simulink model "Copy_of_simpleDemonstrationDouble"  (R2023a)
settings: Solver=VariableStepAuto  StartTime=0.0  StopTime=Tstep*ofdmSymLen*6  RelTol=1e-3
PreLoadFcn:
  | % 100 MHz scenario
  | scs = 30e3;
  | fftLength = 4096;
  | NSubcarriers = 3276;
  | cpLength = 288;
  | windowLength = 20;
  | 
  | nGuardBandCarrier = fftLength - NSubcarriers;
  | ofdmSymLen = fftLength+cpLength;
  | overSamplingRate = 7;
  | filterLength = 6*70;
  | 
  | BW = scs*fftLength;                       %  Signal BW
  | Tstep = 1/BW;                   %  Simulation BW BB
  | RF = 3.7e9;                       %  RF center frequency
  | IF = 500e6;                          % IF frequency
  | dataRatePA = 1/BW;  % PA characterization sample time
  | N = nGuardBandCarrier/2;
  | HPF_cutoff = RF - 500e6;
  | 
  | bw = 100e6;
  | [txWaveform, sampleRate] = helperPACharGenerateOFDM(bw);
  | 
  | dataFileName = sprintf("helperPACharSavedData%dMHz",bw/1e6);
  | load(dataFileName,"results")
  | paInput = results.InputWaveform;
  | paOutput = results.OutputWaveform;
  | modType = 'memPoly';
  | memLen = 5;
  | degLen = 5;
  | halfDataPts = round(length(paInput)/2);
  | origState = warning;
  | warning('off', 'MATLAB:rankDeficientMatrix')
  | paModelMemPoly = double(helperPACharMemPolyModel('coefficientFinder', ...
  |   paInput(1:halfDataPts),paOutput(1:halfDataPts),memLen,degLen,modType));
  | warning(origState);
  | 
  | gain = results.LinearGain;
  | scaleFactor = double(max(abs(paOutput))/max(abs(txWaveform))/gain);
InitFcn:
  | % Initialize model parameters
  | NRInfo = get_param([gcs '/5G NR Test Model'], 'UserData');
  | MultirateBlock = [gcs '/Multirate Parameters'];
  | hInitializeNRTMModel(MultirateBlock,NRInfo);
StopFcn:
  | clear hDecodeSubframe;
undefined symbols (not defined in the file or in its folder): errorPDec, errorPInt, errorStDec, errorStInt, firceqrip, modNFloor, nDec, nInt, OSR, Probability, S, waveform
libraries: simrfV2elements x20, simrfV2util1 x11, simrfV2_lib x5, dspstat3 x4, simrfV2systems x3, commofdm x2, commrfcorlib x2, dspmlti4 x2, simrfV2junction1 x2, commrandsrc3 x1, commdigbbndam3 x1, commutil2 x1
(part 2 of 2)

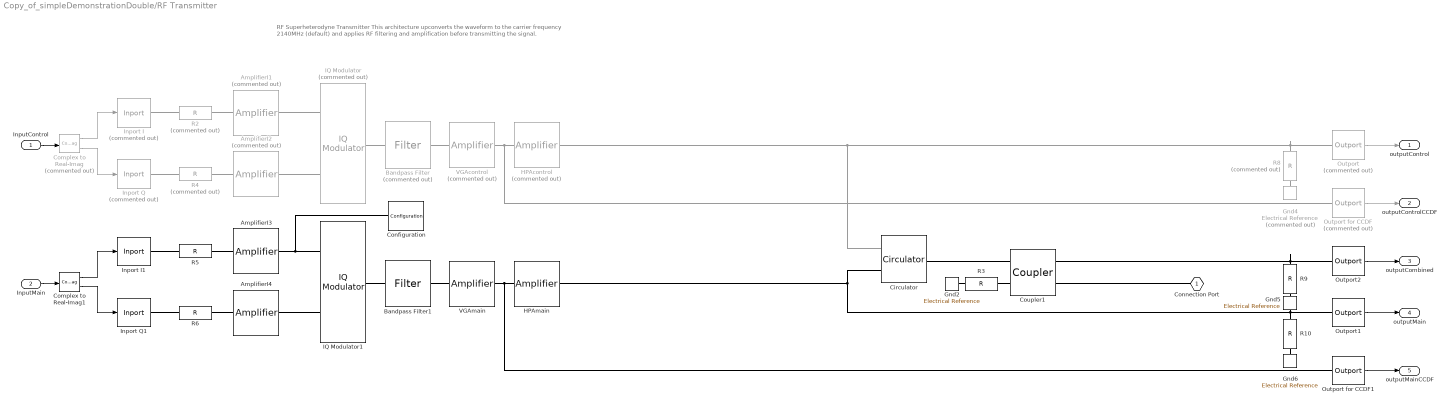
== system Copy_of_simpleDemonstrationDouble/RF Transmitter ==
  note: RF Superheterodyne Transmitter
      |
      | This architecture upconverts the waveform to the carrier frequency 2140MHz (default) and applies RF
      | filtering and amplification before transmitting the signal.
  InputControl : Inport
  InputMain : Inport  Port=2
  AmplifierI1 : simrfV2elements/Amplifier  Commented=on  classname=amplifier  DataSource=Data file  File=unitygain.s2p  isNetworkObj=off  Paramtype=S-parameters  Sparam=[0 0;1 0]  SparamFreq=1e9 Hz  SparamZ0=50  isRationalObj=off  Residues=0  Poles=0  DF={0 0; 1 0}  Source_linear_gain=Available power gain  linear_gain=10*log10(4) dB  AmAmAmPmTable=[-25,5,-1;-10,20,-2;0,27,5;5,28,12]  Zin=50  Zout=50  Source_Poly=Even and odd order  Poly_Coeffs=[0 1]  IPType=Input  IP2=inf dBm  IP3=inf dBm  P1dB=inf dBm  Psat=inf dBm  Gcomp=inf dBm  InternalGrounding=on  SourceFreq=Extracted from data source  PlotFreq=[1e9:1e6:3e9] Hz  PlotType=X-Y plane  YParam1=S(1,1)  YFormat1=Magnitude (dB)  YParam2=None  YFormat2=Magnitude (dB)  YOption=Linear  XOption=Linear  SparamRepresentation=Time domain (rationalfit)  FitTol=-40  FitOpt=Fit individually  MaxPoles=48  AutoImpulseLength=on  ImpulseLength=1e-10 s  MagModeling=off  AddNoise=on  NoiseType=Noise figure  NoiseDist=White  NF=0.2  MinNF=0  Gopt=0  RN=0  CarrierFreq=0 Hz  NoiseAutoImpulseLength=on  NoiseImpulseLength=1e-10 s  ConstS21NL=on  OpFreq=0 Hz  SetOpFreqAsMaxS21=on
  AmplifierI2 : simrfV2elements/Amplifier  Commented=on  classname=amplifier  DataSource=Data file  File=unitygain.s2p  isNetworkObj=off  Paramtype=S-parameters  Sparam=[0 0;1 0]  SparamFreq=1e9 Hz  SparamZ0=50  isRationalObj=off  Residues=0  Poles=0  DF={0 0; 1 0}  Source_linear_gain=Available power gain  linear_gain=10*log10(4) dB  AmAmAmPmTable=[-25,5,-1;-10,20,-2;0,27,5;5,28,12]  Zin=50  Zout=50  Source_Poly=Even and odd order  Poly_Coeffs=[0 1]  IPType=Input  IP2=inf dBm  IP3=inf dBm  P1dB=inf dBm  Psat=inf dBm  Gcomp=inf dBm  InternalGrounding=on  SourceFreq=Extracted from data source  PlotFreq=[1e9:1e6:3e9] Hz  PlotType=X-Y plane  YParam1=S(1,1)  YFormat1=Magnitude (dB)  YParam2=None  YFormat2=Magnitude (dB)  YOption=Linear  XOption=Linear  SparamRepresentation=Time domain (rationalfit)  FitTol=-40  FitOpt=Fit individually  MaxPoles=48  AutoImpulseLength=on  ImpulseLength=1e-10 s  MagModeling=off  AddNoise=on  NoiseType=Noise figure  NoiseDist=White  NF=0.2  MinNF=0  Gopt=0  RN=0  CarrierFreq=0 Hz  NoiseAutoImpulseLength=on  NoiseImpulseLength=1e-10 s  ConstS21NL=on  OpFreq=0 Hz  SetOpFreqAsMaxS21=on
  AmplifierI3 : simrfV2elements/Amplifier  classname=amplifier  DataSource=Data file  File=unitygain.s2p  isNetworkObj=off  Paramtype=S-parameters  Sparam=[0 0;1 0]  SparamFreq=1e9 Hz  SparamZ0=50  isRationalObj=off  Residues=0  Poles=0  DF={0 0; 1 0}  Source_linear_gain=Available power gain  linear_gain=10*log10(4) dB  AmAmAmPmTable=[-25,5,-1;-10,20,-2;0,27,5;5,28,12]  Zin=50  Zout=50  Source_Poly=Even and odd order  Poly_Coeffs=[0 1]  IPType=Input  IP2=inf dBm  IP3=inf dBm  P1dB=inf dBm  Psat=inf dBm  Gcomp=inf dBm  InternalGrounding=on  SourceFreq=Extracted from data source  PlotFreq=[1e9:1e6:3e9] Hz  PlotType=X-Y plane  YParam1=S(1,1)  YFormat1=Magnitude (dB)  YParam2=None  YFormat2=Magnitude (dB)  YOption=Linear  XOption=Linear  SparamRepresentation=Time domain (rationalfit)  FitTol=-40  FitOpt=Fit individually  MaxPoles=48  AutoImpulseLength=on  ImpulseLength=1e-10 s  MagModeling=off  AddNoise=on  NoiseType=Noise figure  NoiseDist=White  NF=0.2  MinNF=0  Gopt=0  RN=0  CarrierFreq=0 Hz  NoiseAutoImpulseLength=on  NoiseImpulseLength=1e-10 s  ConstS21NL=on  OpFreq=0 Hz  SetOpFreqAsMaxS21=on
  AmplifierI4 : simrfV2elements/Amplifier  classname=amplifier  DataSource=Data file  File=unitygain.s2p  isNetworkObj=off  Paramtype=S-parameters  Sparam=[0 0;1 0]  SparamFreq=1e9 Hz  SparamZ0=50  isRationalObj=off  Residues=0  Poles=0  DF={0 0; 1 0}  Source_linear_gain=Available power gain  linear_gain=10*log10(4) dB  AmAmAmPmTable=[-25,5,-1;-10,20,-2;0,27,5;5,28,12]  Zin=50  Zout=50  Source_Poly=Even and odd order  Poly_Coeffs=[0 1]  IPType=Input  IP2=inf dBm  IP3=inf dBm  P1dB=inf dBm  Psat=inf dBm  Gcomp=inf dBm  InternalGrounding=on  SourceFreq=Extracted from data source  PlotFreq=[1e9:1e6:3e9] Hz  PlotType=X-Y plane  YParam1=S(1,1)  YFormat1=Magnitude (dB)  YParam2=None  YFormat2=Magnitude (dB)  YOption=Linear  XOption=Linear  SparamRepresentation=Time domain (rationalfit)  FitTol=-40  FitOpt=Fit individually  MaxPoles=48  AutoImpulseLength=on  ImpulseLength=1e-10 s  MagModeling=off  AddNoise=on  NoiseType=Noise figure  NoiseDist=White  NF=0.2  MinNF=0  Gopt=0  RN=0  CarrierFreq=0 Hz  NoiseAutoImpulseLength=on  NoiseImpulseLength=1e-10 s  ConstS21NL=on  OpFreq=0 Hz  SetOpFreqAsMaxS21=on
  Bandpass Filter : simrfV2elements/Filter  Commented=on  classname=filter  DesignMethod=Chebyshev  ResponseType=Bandpass  Implementation=Transfer function  ImplementationIdeal=Constant per carrier  ImplementationRational=Transfer function  UseFilterOrder=off  FilterOrder=5  PassFreq_lp=1 GHz  PassFreq_hp=2 GHz  PassFreq_bp=bpFilterPassFreq MHz  PassFreq_bs=[1 4] GHz  PassAtten=bpFilterPassAtten  StopFreq_lp=2 GHz  StopFreq_hp=1 GHz  StopFreq_bp=bpFilterStopFreq MHz  StopFreq_bs=[2.1 2.9] GHz  StopAtten=bpFilterStopAtten  Rsrc=bpFilterImpedance  Rload=bpFilterImpedance  AutoImpulseLength=on  ImpulseLength=1e-10 s  InternalGrounding=on  PlotFuncLeft=Voltage transfer  PlotLeftForm=Magnitude (dB)  PlotRightOnVT=None  PlotRightNoTD=None  PlotRightNoGD=None  PlotRightNoIR=None  PlotRightNoSR=None  PlotRightForm=Magnitude (dB)  FreqPoints=logspace(0,10,101)  Freq_unit=Hz  TimePoints=linspace(0,1,1e6+1)  Time_unit=s  XaxisScale=Linear  YaxisScale=Linear  needRedraw=1
  Bandpass Filter1 : simrfV2elements/Filter  classname=filter  DesignMethod=Chebyshev  ResponseType=Bandpass  Implementation=Transfer function  ImplementationIdeal=Constant per carrier  ImplementationRational=Transfer function  UseFilterOrder=off  FilterOrder=5  PassFreq_lp=1 GHz  PassFreq_hp=2 GHz  PassFreq_bp=bpFilterPassFreq MHz  PassFreq_bs=[1 4] GHz  PassAtten=bpFilterPassAtten  StopFreq_lp=2 GHz  StopFreq_hp=1 GHz  StopFreq_bp=bpFilterStopFreq MHz  StopFreq_bs=[2.1 2.9] GHz  StopAtten=bpFilterStopAtten  Rsrc=bpFilterImpedance  Rload=bpFilterImpedance  AutoImpulseLength=on  ImpulseLength=1e-10 s  InternalGrounding=on  PlotFuncLeft=Voltage transfer  PlotLeftForm=Magnitude (dB)  PlotRightOnVT=None  PlotRightNoTD=None  PlotRightNoGD=None  PlotRightNoIR=None  PlotRightNoSR=None  PlotRightForm=Magnitude (dB)  FreqPoints=logspace(0,10,101)  Freq_unit=Hz  TimePoints=linspace(0,1,1e6+1)  Time_unit=s  XaxisScale=Linear  YaxisScale=Linear  needRedraw=1
  Circulator : simrfV2junction1/Circulator  classname=circulators  DataSource=Network-parameters  NumPorts=3  DeviceCirculator=Circulator counter clockwise  DeviceDivider=T power divider  DeviceCoupler=Directional coupler  Paramtype=S-parameters  Sparam=[0 0 1; 1 0 0; 0 1 0]  SparamFreq=1e9 Hz  SparamZ0=50  Phase12=0  Phase33=0  Alpha=0  NumberDividerOutports=2  Coupling=0  Directivity=inf  InsertionLoss=inf  ReturnLoss=inf  InternalGrounding=on  SparamRepresentation=Frequency domain  FitOpt=Share all poles  FitTol=-40  MaxPoles=48
  Complex to Real-Imag : ComplexToRealImag  Commented=on
  Complex to Real-Imag1 : ComplexToRealImag
  Configuration : simrfV2util1/Configuration  AutoFreq=on  Tones="[0.07        2.07] GHz"  Harmonics="[1  3]"  NormalizeCarrierPower=on  SolverType=Auto  UseCCode=on  StepSize=Tstep/overSamplingRate s  AddNoise=on  defaultRNG=on  Seed=0  Temperature=temperature K  SolverDelFlag=0  AbsTol=1e-6  RelTol=1e-3  MaxIter=10  ErrorEstimationType=2-norm over all variables  EnableInterpFilter=off  HiddenFIRfilterControllerParam=off  SmallSignalApprox=off  AllSimFreqs=on  SimFreqs=[] Hz  SimFreqsInternal=[]  SamplesPerFrame=1
  Coupler1 : simrfV2junction1/Coupler  classname=couplers  DataSource=Network-parameters  NumPorts=4  DeviceCirculator=Circulator clockwise  DeviceDivider=T power divider  DeviceCoupler=Directional coupler  Paramtype=S-parameters  Sparam=[0 0 1; 1 0 0; 0 1 0]  SparamFreq=1e9 Hz  SparamZ0=50  Phase12=0  Phase33=0  Alpha=0  NumberDividerOutports=2  Coupling=55  Directivity=inf  InsertionLoss=0.0001  ReturnLoss=inf  InternalGrounding=on  SparamRepresentation=Frequency domain  FitOpt=Share all poles  FitTol=-40  MaxPoles=48
  Gnd2 : simrfV2_lib/Elements/Electrical Reference
      settings: InternalSimscapePortConfiguration="{\"Bottom\":[],\"Left\":[{\"id\":\"V\",\"label\":\"\",\"type\":\"foundation.rf.circuitenvelope\"}],\"Right\":[],\"Top\":[]}"
  Gnd4 : simrfV2_lib/Elements/Electrical Reference  Commented=on
      settings: InternalSimscapePortConfiguration="{\"Bottom\":[],\"Left\":[{\"id\":\"V\",\"label\":\"\",\"type\":\"foundation.rf.circuitenvelope\"}],\"Right\":[],\"Top\":[]}"
  Gnd5 : simrfV2_lib/Elements/Electrical Reference
      settings: InternalSimscapePortConfiguration="{\"Bottom\":[],\"Left\":[{\"id\":\"V\",\"label\":\"\",\"type\":\"foundation.rf.circuitenvelope\"}],\"Right\":[],\"Top\":[]}"
  Gnd6 : simrfV2_lib/Elements/Electrical Reference
      settings: InternalSimscapePortConfiguration="{\"Bottom\":[],\"Left\":[{\"id\":\"V\",\"label\":\"\",\"type\":\"foundation.rf.circuitenvelope\"}],\"Right\":[],\"Top\":[]}"
  HPAcontrol : simrfV2elements/Amplifier  Commented=on  classname=amplifier  DataSource=Network-parameters  File=unitygain.s2p  isNetworkObj=off  Paramtype=S-parameters  Sparam=0  SparamFreq=CarrierFreq GHz  SparamZ0=50  isRationalObj=off  Residues=0  Poles=0  DF={0 0; 1 0}  Source_linear_gain=Available power gain  linear_gain=hpaGain - 3.5 dB  AmAmAmPmTable=[-25,5,-1;-10,20,-2;0,27,5;5,28,12]  Zin=hpaImpedance  Zout=hpaImpedance  Source_Poly=Odd order  Poly_Coeffs=[0 1]  IPType=Output  IP2=inf dBm  IP3=hpaIP3 dBm  P1dB=hpaP1dB dBm  Psat=inf dBm  Gcomp=inf dBm  InternalGrounding=on  SourceFreq=Extracted from data source  PlotFreq=1 Hz  PlotType=X-Y plane  YParam1=S(2,1)  YFormat1=Magnitude (dB)  YParam2=None  YFormat2=Magnitude (dB)  YOption=Linear  XOption=Linear  SparamRepresentation=Frequency domain  FitTol=-40  FitOpt=Fit individually  MaxPoles=48  AutoImpulseLength=off  ImpulseLength=0 s  MagModeling=off  AddNoise=on  NoiseType=Noise figure  NoiseDist=White  NF=hpaNF  MinNF=0  Gopt=0  RN=0  CarrierFreq=0 Hz  NoiseAutoImpulseLength=on  NoiseImpulseLength=1e-10 s  ConstS21NL=on  OpFreq=0 Hz  SetOpFreqAsMaxS21=on
  HPAmain : simrfV2elements/Amplifier  classname=amplifier  DataSource=Network-parameters  File=unitygain.s2p  isNetworkObj=off  Paramtype=S-parameters  Sparam=0  SparamFreq=CarrierFreq GHz  SparamZ0=50  isRationalObj=off  Residues=0  Poles=0  DF={0 0; 1 0}  Source_linear_gain=Available power gain  linear_gain=hpaGain dB  AmAmAmPmTable=[-25,5,-1;-10,20,-2;0,27,5;5,28,12]  Zin=hpaImpedance  Zout=hpaImpedance  Source_Poly=Odd order  Poly_Coeffs=[0 1]  IPType=Output  IP2=inf dBm  IP3=hpaIP3 dBm  P1dB=hpaP1dB dBm  Psat=inf dBm  Gcomp=inf dBm  InternalGrounding=on  SourceFreq=Extracted from data source  PlotFreq=1 Hz  PlotType=X-Y plane  YParam1=S(2,1)  YFormat1=Magnitude (dB)  YParam2=None  YFormat2=Magnitude (dB)  YOption=Linear  XOption=Linear  SparamRepresentation=Frequency domain  FitTol=-40  FitOpt=Fit individually  MaxPoles=48  AutoImpulseLength=off  ImpulseLength=0 s  MagModeling=off  AddNoise=on  NoiseType=Noise figure  NoiseDist=White  NF=hpaNF  MinNF=0  Gopt=0  RN=0  CarrierFreq=0 Hz  NoiseAutoImpulseLength=on  NoiseImpulseLength=1e-10 s  ConstS21NL=on  OpFreq=0 Hz  SetOpFreqAsMaxS21=on
  IQ Modulator : simrfV2systems/IQ Modulator  Commented=on  classname=iqmod  Source_linear_gain=Available power gain  linear_gain=modGain dB  Poly_Coeffs=[0 1]  LOFreq=loFreq MHz  Zin=modImpedance  Zout=modImpedance  AddIRFilters=off  AddCSFilter=off  InternalGrounding=on  ForceNextInit=off  NFloor=modNFloor  GainMismatch=modGainMismatch dB  PhaseMismatch=modPhaseMismatch deg  Isolation=modIsolation dB  AddPhaseNoise=on  PhaseNoiseOffset=modPNOffset  PhaseNoiseLevel=modPNLevel  AutoImpulseLengthPN=off  ImpulseLengthPN=impulseDuration  ImpulseLength_unitPN=s  Source_Poly=Odd order  IPType=Input  IP2=inf dBm  IP3=modIP3 dBm  P1dB=inf dBm  Psat=inf dBm  Gcomp=inf dBm  DesignMethodIR=Ideal  ResponseTypeIR=Lowpass  ImplementationIR=LC Tee  ImplementationIdealIR=Constant per carrier  ImplementationRationalIR=Transfer function  UseFilterOrderIR=on  FilterOrderIR=3  PassFreq_lpIR=1  PassFreq_lp_unitIR=GHz  PassFreq_hpIR=2  PassFreq_hp_unitIR=GHz  PassFreq_bpIR=[2 3]  PassFreq_bp_unitIR=GHz  PassFreq_bsIR=[1 4]  PassFreq_bs_unitIR=GHz  PassAttenIR=10*log10(2)  StopFreq_lpIR=2  StopFreq_lp_unitIR=GHz  StopFreq_hpIR=1  StopFreq_hp_unitIR=GHz  StopFreq_bpIR=[1.5 3.5]  StopFreq_bp_unitIR=GHz  StopFreq_bsIR=[2.1 2.9]  StopFreq_bs_unitIR=GHz  StopAttenIR=40  RsrcIR=50  RloadIR=50  AutoImpulseLengthIR=on  ImpulseLengthIR=1e-10  ImpulseLength_unitIR=s  DesignMethodCS=Ideal  ResponseTypeCS=Highpass  ImplementationCS=LC Tee  ImplementationIdealCS=Constant per carrier  ImplementationRationalCS=Transfer function  UseFilterOrderCS=on  FilterOrderCS=3  PassFreq_lpCS=1  PassFreq_lp_unitCS=GHz  PassFreq_hpCS=2  PassFreq_hp_unitCS=GHz  PassFreq_bpCS=[2 3]  PassFreq_bp_unitCS=GHz  PassFreq_bsCS=[1 4]  PassFreq_bs_unitCS=GHz  PassAttenCS=10*log10(2)  StopFreq_lpCS=2  StopFreq_lp_unitCS=GHz  StopFreq_hpCS=1  StopFreq_hp_unitCS=GHz  StopFreq_bpCS=[1.5 3.5]  StopFreq_bp_unitCS=GHz  StopFreq_bsCS=[2.1 2.9]  StopFreq_bs_unitCS=GHz  StopAttenCS=40  RsrcCS=50  RloadCS=50  AutoImpulseLengthCS=on  ImpulseLengthCS=2.5e-4  ImpulseLength_unitCS=s
  IQ Modulator1 : simrfV2systems/IQ Modulator  classname=iqmod  Source_linear_gain=Available power gain  linear_gain=modGain dB  Poly_Coeffs=[0 1]  LOFreq=loFreq MHz  Zin=modImpedance  Zout=modImpedance  AddIRFilters=off  AddCSFilter=off  InternalGrounding=on  ForceNextInit=off  NFloor=modNFloor  GainMismatch=modGainMismatch dB  PhaseMismatch=modPhaseMismatch deg  Isolation=modIsolation dB  AddPhaseNoise=on  PhaseNoiseOffset=modPNOffset  PhaseNoiseLevel=modPNLevel  AutoImpulseLengthPN=off  ImpulseLengthPN=impulseDuration  ImpulseLength_unitPN=s  Source_Poly=Odd order  IPType=Input  IP2=inf dBm  IP3=modIP3 dBm  P1dB=inf dBm  Psat=inf dBm  Gcomp=inf dBm  DesignMethodIR=Ideal  ResponseTypeIR=Lowpass  ImplementationIR=LC Tee  ImplementationIdealIR=Constant per carrier  ImplementationRationalIR=Transfer function  UseFilterOrderIR=on  FilterOrderIR=3  PassFreq_lpIR=1  PassFreq_lp_unitIR=GHz  PassFreq_hpIR=2  PassFreq_hp_unitIR=GHz  PassFreq_bpIR=[2 3]  PassFreq_bp_unitIR=GHz  PassFreq_bsIR=[1 4]  PassFreq_bs_unitIR=GHz  PassAttenIR=10*log10(2)  StopFreq_lpIR=2  StopFreq_lp_unitIR=GHz  StopFreq_hpIR=1  StopFreq_hp_unitIR=GHz  StopFreq_bpIR=[1.5 3.5]  StopFreq_bp_unitIR=GHz  StopFreq_bsIR=[2.1 2.9]  StopFreq_bs_unitIR=GHz  StopAttenIR=40  RsrcIR=50  RloadIR=50  AutoImpulseLengthIR=on  ImpulseLengthIR=1e-10  ImpulseLength_unitIR=s  DesignMethodCS=Ideal  ResponseTypeCS=Highpass  ImplementationCS=LC Tee  ImplementationIdealCS=Constant per carrier  ImplementationRationalCS=Transfer function  UseFilterOrderCS=on  FilterOrderCS=3  PassFreq_lpCS=1  PassFreq_lp_unitCS=GHz  PassFreq_hpCS=2  PassFreq_hp_unitCS=GHz  PassFreq_bpCS=[2 3]  PassFreq_bp_unitCS=GHz  PassFreq_bsCS=[1 4]  PassFreq_bs_unitCS=GHz  PassAttenCS=10*log10(2)  StopFreq_lpCS=2  StopFreq_lp_unitCS=GHz  StopFreq_hpCS=1  StopFreq_hp_unitCS=GHz  StopFreq_bpCS=[1.5 3.5]  StopFreq_bp_unitCS=GHz  StopFreq_bsCS=[2.1 2.9]  StopFreq_bs_unitCS=GHz  StopAttenCS=40  RsrcCS=50  RloadCS=50  AutoImpulseLengthCS=on  ImpulseLengthCS=2.5e-4  ImpulseLength_unitCS=s
  Inport I : simrfV2util1/Inport  Commented=on  SimulinkInputSignalType=Ideal voltage  CarrierFreq=ifFreq MHz  ZS=0  UseSqWave=off  NumCoeff=10  Bias=0  DutyCyc=50  InternalGrounding=on
  Inport I1 : simrfV2util1/Inport  SimulinkInputSignalType=Ideal voltage  CarrierFreq=ifFreq MHz  ZS=0  UseSqWave=off  NumCoeff=10  Bias=0  DutyCyc=50  InternalGrounding=on
  Inport Q : simrfV2util1/Inport  Commented=on  SimulinkInputSignalType=Ideal voltage  CarrierFreq=ifFreq MHz  ZS=0  UseSqWave=off  NumCoeff=10  Bias=0  DutyCyc=50  InternalGrounding=on
  Inport Q1 : simrfV2util1/Inport  SimulinkInputSignalType=Ideal voltage  CarrierFreq=ifFreq MHz  ZS=0  UseSqWave=off  NumCoeff=10  Bias=0  DutyCyc=50  InternalGrounding=on
  Outport : simrfV2util1/Outport  Commented=on  SensorType=Ideal voltage  OutputFormat=Complex Baseband  CarrierFreq=carrierFreq MHz  ZL=Inf  InternalGrounding=on  StepSize=-1 s  AutoStep=off  HalfPolyphaseLength=0
  Outport for CCDF : simrfV2util1/Outport  Commented=on  SensorType=Ideal voltage  OutputFormat=Complex Baseband  CarrierFreq=carrierFreq MHz  ZL=Inf  InternalGrounding=on  StepSize=-1 s  AutoStep=off  HalfPolyphaseLength=0
  Outport for CCDF1 : simrfV2util1/Outport  SensorType=Ideal voltage  OutputFormat=Complex Baseband  CarrierFreq=carrierFreq MHz  ZL=Inf  InternalGrounding=on  StepSize=-1 s  AutoStep=off  HalfPolyphaseLength=0
  Outport1 : simrfV2util1/Outport  SensorType=Ideal voltage  OutputFormat=Complex Baseband  CarrierFreq=carrierFreq MHz  ZL=Inf  InternalGrounding=on  StepSize=-1 s  AutoStep=off  HalfPolyphaseLength=0
  Outport2 : simrfV2util1/Outport  SensorType=Ideal voltage  OutputFormat=Complex Baseband  CarrierFreq=carrierFreq MHz  ZL=Inf  InternalGrounding=on  StepSize=-1 s  AutoStep=off  HalfPolyphaseLength=0
  R{3,5..6,9..10} (5 alike) : simrfV2elements/R  classname=resistor  Resistance=50 Ohm  AddNoise=on
  R2 : simrfV2elements/R  Commented=on  classname=resistor  Resistance=50 Ohm  AddNoise=on
  R4 : simrfV2elements/R  Commented=on  classname=resistor  Resistance=50 Ohm  AddNoise=on
  R8 : simrfV2elements/R  Commented=on  classname=resistor  Resistance=50 Ohm  AddNoise=on
  VGAcontrol : simrfV2elements/Amplifier  Commented=on  classname=amplifier  DataSource=Network-parameters  File=unitygain.s2p  isNetworkObj=off  Paramtype=S-parameters  Sparam=0  SparamFreq=CarrierFreq GHz  SparamZ0=50  isRationalObj=off  Residues=0  Poles=0  DF={0 0; 1 0}  Source_linear_gain=Available power gain  linear_gain=vgaGain dB  AmAmAmPmTable=[-25,5,-1;-10,20,-2;0,27,5;5,28,12]  Zin=vgaImpedance  Zout=vgaImpedance  Source_Poly=Odd order  Poly_Coeffs=[0 1]  IPType=Output  IP2=inf dBm  IP3=vgaIP3 dBm  P1dB=vgaP1dB dBm  Psat=inf dBm  Gcomp=inf dBm  InternalGrounding=on  SourceFreq=Extracted from data source  PlotFreq=1 Hz  PlotType=X-Y plane  YParam1=S(2,1)  YFormat1=Magnitude (dB)  YParam2=None  YFormat2=Magnitude (dB)  YOption=Linear  XOption=Linear  SparamRepresentation=Frequency domain  FitTol=-40  FitOpt=Fit individually  MaxPoles=48  AutoImpulseLength=off  ImpulseLength=0 s  MagModeling=off  AddNoise=on  NoiseType=Noise figure  NoiseDist=White  NF=vgaNF  MinNF=0  Gopt=0  RN=0  CarrierFreq=0 Hz  NoiseAutoImpulseLength=on  NoiseImpulseLength=1e-10 s  ConstS21NL=on  OpFreq=0 Hz  SetOpFreqAsMaxS21=on
  VGAmain : simrfV2elements/Amplifier  classname=amplifier  DataSource=Network-parameters  File=unitygain.s2p  isNetworkObj=off  Paramtype=S-parameters  Sparam=0  SparamFreq=CarrierFreq GHz  SparamZ0=50  isRationalObj=off  Residues=0  Poles=0  DF={0 0; 1 0}  Source_linear_gain=Available power gain  linear_gain=vgaGain dB  AmAmAmPmTable=[-25,5,-1;-10,20,-2;0,27,5;5,28,12]  Zin=vgaImpedance  Zout=vgaImpedance  Source_Poly=Odd order  Poly_Coeffs=[0 1]  IPType=Output  IP2=inf dBm  IP3=vgaIP3 dBm  P1dB=vgaP1dB dBm  Psat=inf dBm  Gcomp=inf dBm  InternalGrounding=on  SourceFreq=Extracted from data source  PlotFreq=1 Hz  PlotType=X-Y plane  YParam1=S(2,1)  YFormat1=Magnitude (dB)  YParam2=None  YFormat2=Magnitude (dB)  YOption=Linear  XOption=Linear  SparamRepresentation=Frequency domain  FitTol=-40  FitOpt=Fit individually  MaxPoles=48  AutoImpulseLength=off  ImpulseLength=0 s  MagModeling=off  AddNoise=on  NoiseType=Noise figure  NoiseDist=White  NF=vgaNF  MinNF=0  Gopt=0  RN=0  CarrierFreq=0 Hz  NoiseAutoImpulseLength=on  NoiseImpulseLength=1e-10 s  ConstS21NL=on  OpFreq=0 Hz  SetOpFreqAsMaxS21=on
  Connection Port : PMIOPort  Tag=simrfV2util1/Connection Port  Side=Right
  outputControl : Outport
  outputControlCCDF : Outport  Port=2
  outputCombined : Outport  Port=3
  outputMain : Outport  Port=4
  outputMainCCDF : Outport  Port=5
  wires:
  Complex to Real-Imag/1 -> Inport I/1
  Complex to Real-Imag/2 -> Inport Q/1
  Outport/1 -> outputControl/1
  InputControl/1 -> Complex to Real-Imag/1
  Outport for CCDF/1 -> outputControlCCDF/1
  InputMain/1 -> Complex to Real-Imag1/1
  Outport for CCDF1/1 -> outputMainCCDF/1
  Outport1/1 -> outputMain/1
  Complex to Real-Imag1/2 -> Inport Q1/1
  Complex to Real-Imag1/1 -> Inport I1/1
  Outport2/1 -> outputCombined/1
  connections:
  Bandpass Filter/LConn1 -- IQ Modulator/RConn1
  Bandpass Filter/RConn1 -- VGAcontrol/LConn1
  HPAcontrol/LConn1 -- Outport for CCDF/LConn1 -- VGAcontrol/RConn1
  HPAcontrol/RConn1 -- Circulator/LConn1 -- R8/LConn1 -- Outport/LConn1
  VGAmain/RConn1 -- Outport for CCDF1/LConn1 -- HPAmain/LConn1
  Bandpass Filter1/RConn1 -- VGAmain/LConn1
  HPAmain/RConn1 -- Circulator/LConn2 -- R10/LConn1 -- Outport1/LConn1
  AmplifierI1/RConn1 -- IQ Modulator/LConn1
  R2/LConn1 -- Inport I/RConn1
  AmplifierI1/LConn1 -- R2/RConn1
  R4/LConn1 -- Inport Q/RConn1
  AmplifierI2/LConn1 -- R4/RConn1
  AmplifierI4/RConn1 -- IQ Modulator1/LConn2
  AmplifierI3/RConn1 -- Configuration/LConn1 -- IQ Modulator1/LConn1
  AmplifierI4/LConn1 -- R6/RConn1
  Inport Q1/RConn1 -- R6/LConn1
  IQ Modulator1/RConn1 -- Bandpass Filter1/LConn1
  Inport I1/RConn1 -- R5/LConn1
  AmplifierI3/LConn1 -- R5/RConn1
  R3/LConn1 -- Coupler1/LConn2
  Gnd2/LConn1 -- R3/RConn1
  Circulator/RConn1 -- Coupler1/LConn1
  Coupler1/RConn1 -- R9/LConn1 -- Outport2/LConn1
  Coupler1/RConn2 -- Connection Port/RConn1
  R8/RConn1 -- Gnd4/LConn1
  R9/RConn1 -- Gnd5/LConn1
  R10/RConn1 -- Gnd6/LConn1
  AmplifierI2/RConn1 -- IQ Modulator/LConn2

== matlab function Copy_of_simpleDemonstrationDouble/5G NR Test Model ==
  data: wf output; waveform parameter; nsamps parameter; OutputAfterFinalValue parameter
function wf = wfGenerator(waveform, nsamps, OutputAfterFinalValue)

% Create persistent variable
persistent src;

% Preallocate output
wf = complex(zeros(nsamps,size(waveform,2)));

if isempty(src)
    % Get action when signal ends
    if OutputAfterFinalValue == 1
        signalEndAction = 'Cyclic repetition';
    else
        signalEndAction = 'Set to zero';
    end
    
    % Initialize persistent dsp.SignalSource to get current frame
    src = dsp.SignalSource(waveform,nsamps,'SignalEndAction',signalEndAction);
end

% Extract current frame
wf(:,:) = src();

end

== matlab function Copy_of_simpleDemonstrationDouble/Calculate TX EVM/MATLAB Function ==
  data: rxSig input; scaledSig output; ref input; gain output
function [scaledSig, gain] = scaleRotate(rxSig,ref)
persistent c
persistent invCov
if isempty(c)
    c = complex(ones(size(rxSig)));
end
if isempty(invCov)
    invCov = complex(ones(size(rxSig)));
end

scaledSig = c.*rxSig;
errsig = ref - scaledSig;

% RLS algorithm
lambda = 0.99;
XP = conj(rxSig).*invCov;
invDen = 1./(lambda + XP.*rxSig);
K = invDen.*(invCov.*rxSig);
invCov = (1/lambda)*(invCov - K.*XP);
c = c + errsig .* conj(K);

gain = c;

== matlab function Copy_of_simpleDemonstrationDouble/Decode Subframe ==
  data: EVM output; pdschSym output size=NRInfo.WaveformLength; subframe input; EVM3GPP parameter
%hDecodeSf Subframe decodification and EVM calculation
%   [EVM,PDSCHSYM] = hDecodeSf(SUBFRAME) calls the function which decodes
%   the subframe SUBFRAME. It returns the decoded symbols
%   PDSCHSYM and the average EVM.

%   Copyright 2019-2021 The MathWorks, Inc.

function [EVM,pdschSym] = hDecodeSf(subframe,EVM3GPP)

    coder.extrinsic('hDecodeSubframe');

    % Create count to track number of current transmitted subframe
    persistent count; 
    
    % Create persistent variables for current and previous subframes
    persistent subframe1
    persistent subframe2

    % Specify output type
    pdschSym = complex(0,0); 
    EVM = 0; %#ok<NASGU>

    % Initialize the persistent variables
    if isempty(count)
        count = -2; 
        subframe2 = subframe;
        subframe1 = 0;
        subframes = 0;
    else
        subframe1 = subframe2;
        subframe2 = subframe;
        subframes = [subframe1; subframe2];
    end

    % Get the number of the current transmitted subframe
    numberFrames = 10;
    subframeNo = mod(double(count),numberFrames);
    
    % Decode a length of two subframes to account for time delays
    if count > -1
        [evm,pdschsym]  = hDecodeSubframe(subframeNo,subframes,count,EVM3GPP);
        pdschSym(:) = pdschsym;
        EVM = evm;
    else
        pdschSym(:) = NaN;
        EVM = NaN;
    end

    % Increment counter
    count = count + 1;

end
